simulink model "Test_Decoder_5_to_32"  (Simulink 8.7)
settings: Solver=ode45  StartTime=0.0  StopTime=len  RelTol=1e-3
libraries: commutil2 x2, Decoders_Lib x1
settings Model: Creator=N  LastModifiedBy=Jozko Mrkvicka
settings DataIOCC: LimitDataPoints=off
settings DebuggingCC: UnderspecifiedInitializationDetection=Simplified  MergeDetectMultiDrivingBlocksExec=error
settings HardwareCC: ProdBitPerPointer=64  ProdLargestAtomicFloat=Float  ProdIntDivRoundTo=Zero  ProdEndianess=LittleEndian  ProdHWDeviceType=Intel->x86-64 (Windows64)
settings ModelReferenceCC: PropagateSignalLabelsOutOfModel=on

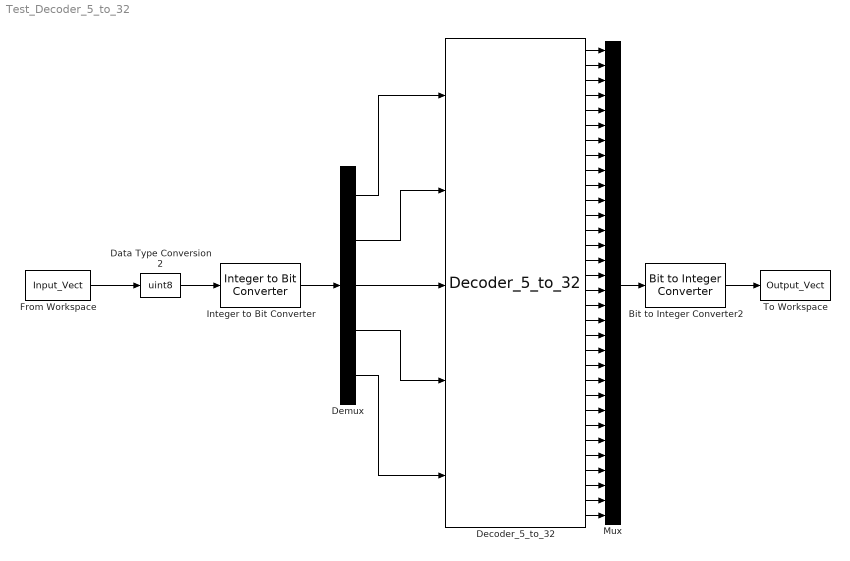
== system Test_Decoder_5_to_32 ==
  Bit to Integer Converter2 : commutil2/Bit to Integer Converter  nbits=32  bitOrder=MSB first  signedOutputValues=Unsigned  outDtype=uint32  outDtypeSigned=Inherit via internal rule
  Data Type Conversion2 : DataTypeConversion  OutDataTypeStr=uint8
  Decoder_5_to_32 : Decoders_Lib/Decoders_Lib/Decoder_5_to_32
  Demux : Demux  Outputs=5
  From Workspace : FromWorkspace  VariableName=Input_Vect  SampleTime=1  Interpolate=off  OutputAfterFinalValue=Holding final value
  Integer to Bit Converter : commutil2/Integer to Bit Converter  nbits=5  signedInputValues=Unsigned  bitOrder=MSB first  outDtype=uint8
  Mux : Mux  Inputs=32
  To Workspace : ToWorkspace  VariableName=Output_Vect  SampleTime=1
  wires:
  Integer to Bit Converter/1 -> Demux/1
  Data Type Conversion2/1 -> Integer to Bit Converter/1
  Mux/1 -> Bit to Integer Converter2/1
  From Workspace/1 -> Data Type Conversion2/1
  Bit to Integer Converter2/1 -> To Workspace/1
  Decoder_5_to_32/1 -> Mux/1
  Decoder_5_to_32/2 -> Mux/2
  Decoder_5_to_32/3 -> Mux/3
  Decoder_5_to_32/4 -> Mux/4
  Decoder_5_to_32/5 -> Mux/5
  Decoder_5_to_32/6 -> Mux/6
  Decoder_5_to_32/7 -> Mux/7
  Decoder_5_to_32/8 -> Mux/8
  Decoder_5_to_32/9 -> Mux/9
  Decoder_5_to_32/10 -> Mux/10
  Decoder_5_to_32/11 -> Mux/11
  Decoder_5_to_32/12 -> Mux/12
  Decoder_5_to_32/13 -> Mux/13
  Decoder_5_to_32/14 -> Mux/14
  Decoder_5_to_32/15 -> Mux/15
  Decoder_5_to_32/16 -> Mux/16
  Decoder_5_to_32/17 -> Mux/17
  Decoder_5_to_32/18 -> Mux/18
  Decoder_5_to_32/19 -> Mux/19
  Decoder_5_to_32/20 -> Mux/20
  Decoder_5_to_32/21 -> Mux/21
  Decoder_5_to_32/22 -> Mux/22
  Decoder_5_to_32/23 -> Mux/23
  Decoder_5_to_32/24 -> Mux/24
  Decoder_5_to_32/25 -> Mux/25
  Decoder_5_to_32/26 -> Mux/26
  Decoder_5_to_32/27 -> Mux/27
  Decoder_5_to_32/28 -> Mux/28
  Decoder_5_to_32/29 -> Mux/29
  Decoder_5_to_32/30 -> Mux/30
  Decoder_5_to_32/31 -> Mux/31
  Decoder_5_to_32/32 -> Mux/32
  Demux/3 -> Decoder_5_to_32/3
  Demux/2 -> Decoder_5_to_32/2
  Demux/1 -> Decoder_5_to_32/1
  Demux/4 -> Decoder_5_to_32/4
  Demux/5 -> Decoder_5_to_32/5
